simulink model "Complete"  (R2019b)
settings: Solver=ode45  StartTime=0.0  StopTime=0.5  RelTol=1e-3  EnableMultiTasking=on
InitFcn:
  | load_from_scope
values from neighbouring files (symbols this model uses):
  dt = double(convertCharsToStrings(char(dt(1:end-1))))    [load_from_scope.m]
libraries: DTMFLibrary x9
settings Model: Creator=eeguest  LastModifiedBy=zceeash
settings DataIOCC: LimitDataPoints=on  SaveFormat=Array  SignalLoggingSaveFormat=ModelDataLogs  ReturnWorkspaceOutputs=off
settings OptimizationCC: ExpressionDepthLimit=2147483647  LifeSpan=inf
settings DebuggingCC: UnderspecifiedInitializationDetection=Classic  MergeDetectMultiDrivingBlocksExec=none  SolverPrmCheckMsg=warning  FcnCallInpInsideContextMsg=warning  StateNameClashWarn=warning  SFUnexpectedBacktrackingDiag=warning  SFNoUnconditionalDefaultTransitionDiag=warning  SFExecutionAtInitializationDiag=none  ArithmeticOperatorsInVariantConditions=warning
settings HardwareCC: ProdBitPerPointer=32  ProdBitPerSizeT=32  ProdBitPerPtrDiffT=32  ProdLargestAtomicFloat=None  ProdIntDivRoundTo=Undefined  ProdEndianess=Unspecified  ProdWordSize=32  ProdHWDeviceType=32-bit Generic
settings ModelReferenceCC: PropagateSignalLabelsOutOfModel=off
settings SFSimCC: SimUseLocalCustomCode=off  CustomCodeUndefinedFunction=UseInterfaceOnly
settings RTWCC: RTWUseLocalCustomCode=off
settings CodeAppCC: StateflowObjectComments=on
settings GRTTargetCC: TargetLangStandard=C89/C90 (ANSI)  GeneratePreprocessorConditionals=Disable all
settings ConfigComp: CovMetricSettings=dw  CovHtmlReporting=on  CovSaveCumulativeToWorkspaceVar=on  CovSaveSingleToWorkspaceVar=on  CovExternalEMLEnable=off  CovSFcnEnable=off

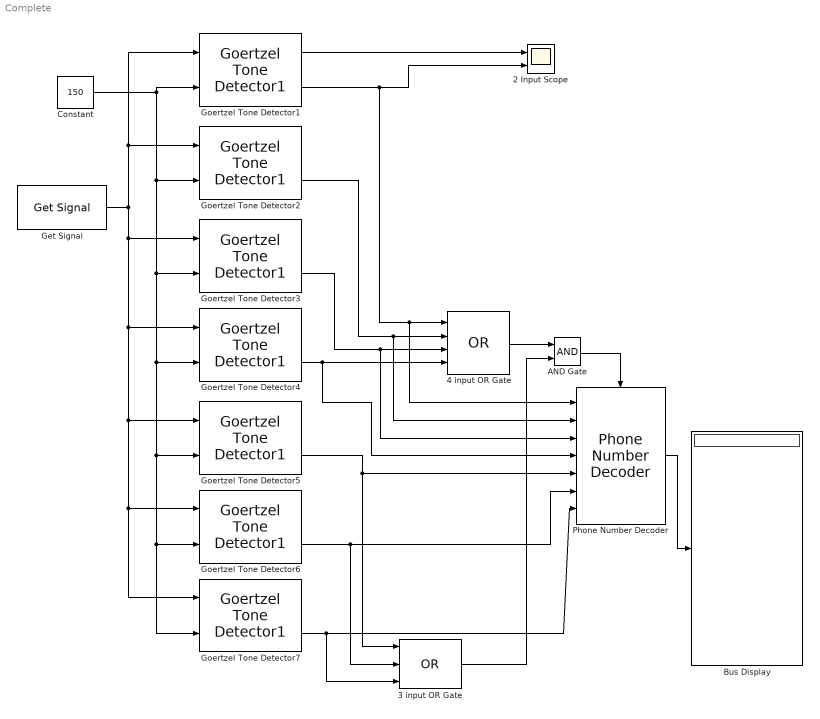
== system Complete ==
  2 Input Scope : Scope  NumInputPorts=2
  3 input OR Gate : Logic  Operator=OR  Inputs=3  AllPortsSameDT=off  OutDataTypeStr=boolean
  4 input OR Gate : Logic  Operator=OR  Inputs=4  AllPortsSameDT=off  OutDataTypeStr=boolean
  AND Gate : Logic  AllPortsSameDT=off  OutDataTypeStr=boolean
  Bus Display : Display
  Constant : Constant  Value=150
  Get Signal : DTMFLibrary/Get Signal  VariableName=data_matrix  SampleTime=dt  OutputAfterFinalValue=Setting to zero
  Goertzel Tone Detector1 : DTMFLibrary/Goertzel Tone Detector1  ToneFreq=697  EstWindow=0.01
  Goertzel Tone Detector2 : DTMFLibrary/Goertzel Tone Detector1  ToneFreq=770  EstWindow=0.01
  Goertzel Tone Detector3 : DTMFLibrary/Goertzel Tone Detector1  ToneFreq=852  EstWindow=0.01
  Goertzel Tone Detector4 : DTMFLibrary/Goertzel Tone Detector1  ToneFreq=941  EstWindow=0.01
  Goertzel Tone Detector5 : DTMFLibrary/Goertzel Tone Detector1  ToneFreq=1209  EstWindow=0.01
  Goertzel Tone Detector6 : DTMFLibrary/Goertzel Tone Detector1  ToneFreq=1336  EstWindow=0.01
  Goertzel Tone Detector7 : DTMFLibrary/Goertzel Tone Detector1  ToneFreq=1477  EstWindow=0.01
  Phone Number Decoder : DTMFLibrary/Phone Number Decoder
  wires:
  Get Signal/1 -> Goertzel Tone Detector2/1, Goertzel Tone Detector1/1, Goertzel Tone Detector4/1, Goertzel Tone Detector5/1, Goertzel Tone Detector6/1, Goertzel Tone Detector7/1, Goertzel Tone Detector3/1
  Constant/1 -> Goertzel Tone Detector1/2, Goertzel Tone Detector2/2, Goertzel Tone Detector3/2, Goertzel Tone Detector4/2, Goertzel Tone Detector5/2, Goertzel Tone Detector6/2, Goertzel Tone Detector7/2
  Goertzel Tone Detector1/1 -> 2 Input Scope/1
  Goertzel Tone Detector1/2 -> Phone Number Decoder/1, 4 input OR Gate/1, 2 Input Scope/2
  Goertzel Tone Detector5/2 -> Phone Number Decoder/5, 3 input OR Gate/1
  Goertzel Tone Detector6/2 -> Phone Number Decoder/6, 3 input OR Gate/2
  Goertzel Tone Detector4/2 -> Phone Number Decoder/4, 4 input OR Gate/4
  Goertzel Tone Detector3/2 -> Phone Number Decoder/3, 4 input OR Gate/3
  Goertzel Tone Detector2/2 -> Phone Number Decoder/2, 4 input OR Gate/2
  3 input OR Gate/1 -> AND Gate/2
  4 input OR Gate/1 -> AND Gate/1
  Goertzel Tone Detector7/2 -> Phone Number Decoder/7, 3 input OR Gate/3
  AND Gate/1 -> Phone Number Decoder/Trigger
  Phone Number Decoder/1 -> Bus Display/1
